simulink model "Model"  (R2023b)
settings: Solver=VariableStepAuto  StartTime=0.0  StopTime=1  RelTol=1e-3
undefined symbols (not defined in the file): D1, Delta
libraries: spsThreePhaseTransformerTwoWindingsLib x4, spsThreePhaseProgrammableVoltageSourceLib x2, spsGroundLib x2, spsDistributedParametersLineLib x2, spsThreePhaseMutualInductanceZ1Z0Lib x2, spsThreePhaseFaultLib x1, spsThreePhaseParallelRLCLoadLib x1, spsThreePhaseVIMeasurementLib x1, sps_lib x1
settings Model: Creator=SJ  LastModifiedBy=SJ

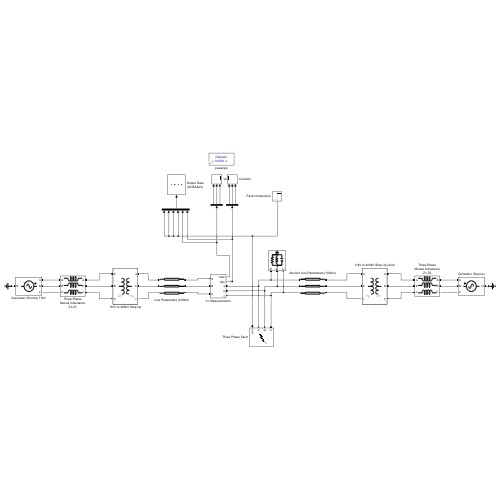
[thumbnail: Simulink's stored preview of the top-level diagram]
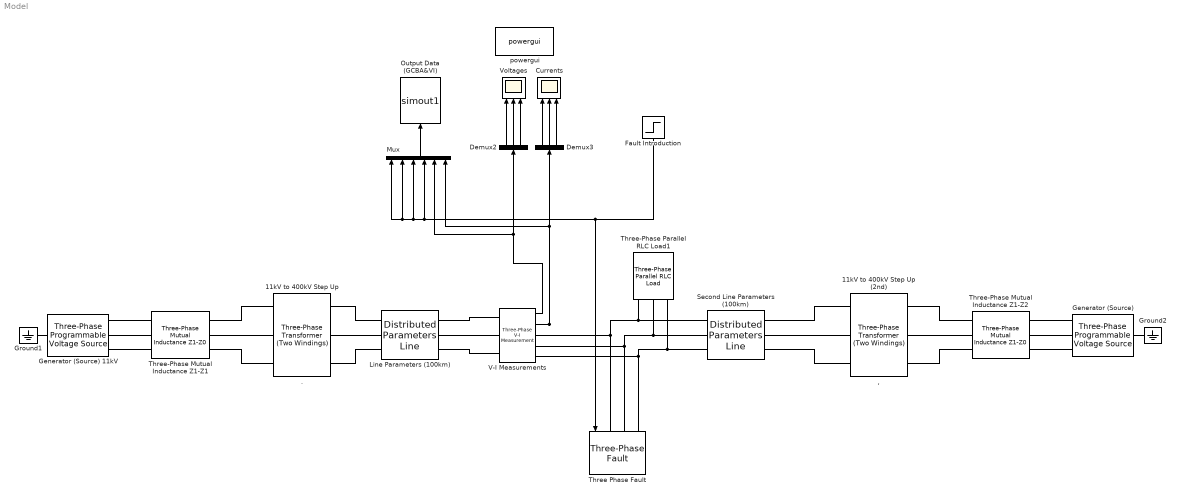
== system Model ==
  , : spsThreePhaseTransformerTwoWindingsLib/Three-Phase Transformer (Two Windings)  Winding1Connection=Delta (D1)  Winding2Connection=Yg  CoreType=Three single-phase transformers  SetSaturation=off  Hysteresis=off  DataFile='hysteresis'  SetInitialFlux=off  Measurements=None  UNITS=pu  NominalPower=[ 2500e3 , 50 ]  Winding1=[ 11e3 , 0.002 , 0.08 ]  Winding2=[ 4e5, 0.002, 0.08 ]  Rm=500  Lm=500  L0=0.5  Saturation=[ 0,0 ; 0.0024,1.2 ; 1.0,1.52 ]  InitialFluxes=[ 0.8 , -0.8 , 0.7 ]  BreakLoop=off  DiscreteSolver=Trapezoidal iterative  DataType=off  TransfoNumber=1
  . : spsThreePhaseTransformerTwoWindingsLib/Three-Phase Transformer (Two Windings)  Winding1Connection=Delta (D1)  Winding2Connection=Yg  CoreType=Three single-phase transformers  SetSaturation=off  Hysteresis=off  DataFile='hysteresis'  SetInitialFlux=off  Measurements=None  UNITS=pu  NominalPower=[ 2500e3 , 50 ]  Winding1=[ 11e3 , 0.002 , 0.08 ]  Winding2=[ 4e5, 0.002, 0.08 ]  Rm=500  Lm=500  L0=0.5  Saturation=[ 0,0 ; 0.0024,1.2 ; 1.0,1.52 ]  InitialFluxes=[ 0.8 , -0.8 , 0.7 ]  BreakLoop=off  DiscreteSolver=Trapezoidal iterative  DataType=off  TransfoNumber=1
  11kV to 400kV Step Up : spsThreePhaseTransformerTwoWindingsLib/Three-Phase Transformer (Two Windings)  Winding1Connection=Delta (D1)  Winding2Connection=Yg  CoreType=Three single-phase transformers  SetSaturation=off  Hysteresis=off  DataFile='hysteresis'  SetInitialFlux=off  Measurements=None  UNITS=pu  NominalPower=[ 2500e3 , 50 ]  Winding1=[ 11e3 , 0.002 , 0.08 ]  Winding2=[ 4e2, 0.002, 0.08 ]  Rm=500  Lm=500  L0=0.5  Saturation=[ 0,0 ; 0.0024,1.2 ; 1.0,1.52 ]  InitialFluxes=[ 0.8 , -0.8 , 0.7 ]  BreakLoop=off  DiscreteSolver=Trapezoidal iterative  DataType=off  TransfoNumber=1
  11kV to 400kV Step Up (2nd) : spsThreePhaseTransformerTwoWindingsLib/Three-Phase Transformer (Two Windings)  Winding1Connection=Delta (D1)  Winding2Connection=Yg  CoreType=Three single-phase transformers  SetSaturation=off  Hysteresis=off  DataFile='hysteresis'  SetInitialFlux=off  Measurements=None  UNITS=pu  NominalPower=[ 2500e3 , 50 ]  Winding1=[ 11e3 , 0.002 , 0.08 ]  Winding2=[ 4e2 , 0.002 , 0.08 ]  Rm=500  Lm=500  L0=0.5  Saturation=[ 0,0 ; 0.0024,1.2 ; 1.0,1.52 ]  InitialFluxes=[ 0.8 , -0.8 , 0.7 ]  BreakLoop=off  DiscreteSolver=Trapezoidal iterative  DataType=off  TransfoNumber=1
  Currents : Scope  NumInputPorts=3
  Demux2 : Demux  Outputs=3
  Demux3 : Demux  Outputs=3
  Fault Introduction : Step  Time=0.1  SampleTime=0
  Generator (Source) : spsThreePhaseProgrammableVoltageSourceLib/Three-Phase Programmable Voltage Source  PositiveSequence="[11e3  0 50]"  VariationEntity=None  VariationType=Table of time-amplitude pairs  VariationTypeAlt=Step  VariationStep=0.5  VariationRate=10  VariationMagnitude=0.3  VariationFrequency=2  VariationTiming=[1 2]  VariationPhaseA=off  Amplitudes=[1 0.8 1.2 1.0]  TimeValues=[0 0.1 0.15 0.2]  HarmonicGeneration=off  HarmonicA=[3 0.2 -25 0]  HarmonicB=[2 0.15 35 2]  Timing="[0.05  3]"  BusType=swing  Pref=0  Qref=0  Qmin=-inf  Qmax=inf
  Generator (Source) 11kV : spsThreePhaseProgrammableVoltageSourceLib/Three-Phase Programmable Voltage Source  PositiveSequence="[11e3  0 50]"  VariationEntity=None  VariationType=Table of time-amplitude pairs  VariationTypeAlt=Step  VariationStep=0.5  VariationRate=10  VariationMagnitude=0.3  VariationFrequency=2  VariationTiming=[1 2]  VariationPhaseA=off  Amplitudes=[1 0.8 1.2 1.0]  TimeValues=[0 0.1 0.15 0.2]  HarmonicGeneration=off  HarmonicA=[3 0.2 -25 0]  HarmonicB=[2 0.15 35 2]  Timing="[0.05  3]"  BusType=swing  Pref=0  Qref=0  Qmin=-inf  Qmax=inf
  Ground1 : spsGroundLib/Ground  LConnTagsString=a
  Ground2 : spsGroundLib/Ground  LConnTagsString=a
  Line Parameters (100km) : spsDistributedParametersLineLib/Distributed Parameters Line  Phases=3  Length=100  Frequency=50  Resistance=[0.01273 0.3864]  Inductance="[0.9337e-3  4.1264e-3]"  Capacitance=[12.74e-9 7.751e-9]  x1=[-0.0006 -4.82329263048478e-14 302.291329147411 -261.391829825195;-0.0005 -4.02670460526195e-14 310.352682416144 -251.767648625029;-0.0004 -3.22614270874366e-14 318.107755056666 -241.895003151946;-0.0003 -2.42239699886876e-14 325.548893748562 -231.78363651509;-0.0002 -1.61626067561552e-14 332.668754986322 -221.443527412571;-0.0001 -8.08529298208965e-15 339.460312326496 -210.884880283698]  x2=[-0.0006 1.07075587974401e-13 258.197390789364 -298.948014119863;-0.0005 1.01302421932401e-13 267.460170011688 -290.690325284424;-0.0004 9.54292826303437e-14 276.458998337068 -282.145760193398;-0.0003 8.94619661476469e-14 285.184995008388 -273.322751300931;-0.0002 8.34063615052364e-14 293.629548520437 -264.230005851586;-0.0001 7.72684448537924e-14 301.784325118421 -254.876497287341]  x3=[-0.0006 3.2797979396176e-15 -0.28191137078804 0.421950096006032;-0.0005 3.29091704997219e-15 -0.295026037352981 0.412886838955771;-0.0004 3.2987884225157e-15 -0.307849548837979 0.403416112443893;-0.0003 3.30340428915374e-15 -0.320369249985401 0.393547262934051;-0.0002 3.30476009458321e-15 -0.332572785361736 0.383290029789229;-0.0001 3.30285450078786e-15 -0.344448111550917 0.372654535660172]  x4=[-0.0006 -3.17636211581e-15 2.23300549703812 -2.5964882734215;-0.0005 -3.15925327302886e-15 2.31346131122797 -2.52506666550988;-0.0004 -3.13902662868852e-15 2.39163401841121 -2.45115312165439;-0.0003 -3.11570214404494e-15 2.46744647156375 -2.37482058559914;-0.0002 -3.08930283754847e-15 2.54082385294727 -2.29614438834146;-0.0001 -3.05985476212738e-15 2.61169374794533 -2.21520217378936]  x5=0.000565541566995743  V1=[2.024e-13 399.6 399.6;314.2 314.2 314.2;-1.932 0.938 -0.6328]  V2=[2.05e-13 395 395;314.2 314.2 314.2;0.8051 0.7925 -0.7783]  I1=[3.039e-15 0.5075 0.5075;314.2 314.2 314.2;-0.08862 -2.472 2.24]  I2=[2.819e-15 3.425 3.425;314.2 314.2 314.2;3.041 0.7904 -0.7804]  nHarmo=1  Measurements=None  Decoupling=off  VsMag0=0  VrMag0=0  VsAngle0=0  VrAngle0=0  IsMag0=0  IrMag0=0  IsAngle0=0  IrAngle0=0
      settings: LibrarySourceBlock=sps_lib/Power Grid Elements/Distributed Parameters Line
  Mux : Mux  Inputs=6
  Output Data (GCBA&VI) : ToWorkspace  VariableName=simout1  SaveFormat=Timeseries  SampleTime=-1
  Second Line Parameters (100km) : spsDistributedParametersLineLib/Distributed Parameters Line  Phases=3  Length=100  Frequency=60  Resistance=[0.01273 0.3864]  Inductance="[0.9337e-3  4.1264e-3]"  Capacitance=[12.74e-9 7.751e-9]  x1=[-0.0006 -1.36928565449085e-13 302.291329147411 -261.391829825195;-0.0005 -1.38135887665828e-13 310.352682416144 -251.767648625028;-0.0004 -1.39206886438792e-13 318.107755056666 -241.895003151946;-0.0003 -1.40140504821492e-13 325.548893748562 -231.78363651509;-0.0002 -1.40935821445302e-13 332.668754986322 -221.443527412571;-0.0001 -1.41592051428733e-13 339.460312326496 -210.884880283698]  x2=[-0.0006 1.07075587974401e-13 258.197390789364 -298.948014119863;-0.0005 1.01302421932401e-13 267.460170011688 -290.690325284424;-0.0004 9.54292826303437e-14 276.458998337068 -282.145760193398;-0.0003 8.94619661476469e-14 285.184995008388 -273.322751300931;-0.0002 8.34063615052364e-14 293.629548520437 -264.230005851586;-0.0001 7.72684448537924e-14 301.784325118421 -254.876497287341]  x3=[-0.0006 1.12667629661657e-15 -0.281911370788044 0.421950096006022;-0.0005 1.11731299989936e-15 -0.295026037352985 0.412886838955761;-0.0004 1.10684705014609e-15 -0.307849548837983 0.403416112443883;-0.0003 1.09528877598558e-15 -0.320369249985405 0.39354726293404;-0.0002 1.082649584039e-15 -0.332572785361739 0.383290029789218;-0.0001 1.06894194766283e-15 -0.34444811155092 0.37265453566016]  x4=[-0.0006 -3.19598852625168e-15 2.23300549703812 -2.59648827342149;-0.0005 -3.24813563146854e-15 2.31346131122797 -2.52506666550987;-0.0004 -3.2970772189693e-15 2.39163401841121 -2.45115312165439;-0.0003 -3.34276498931591e-15 2.46744647156374 -2.37482058559913;-0.0002 -3.38515385419496e-15 2.54082385294727 -2.29614438834145;-0.0001 -3.4242019809145e-15 2.61169374794533 -2.21520217378935]  x5=0.000565541566995742  V1=[3.558e-13 399.6 399.6;314.2 314.2 314.2;-1.251 0.938 -0.6328]  V2=[2.05e-13 395 395;314.2 314.2 314.2;0.8051 0.7925 -0.7783]  I1=[4.38e-15 0.5075 0.5075;314.2 314.2 314.2;0.2418 -2.472 2.24]  I2=[2.604e-15 3.425 3.425;314.2 314.2 314.2;-2.475 0.7904 -0.7804]  nHarmo=1  Measurements=None  Decoupling=off  VsMag0=0  VrMag0=0  VsAngle0=0  VrAngle0=0  IsMag0=0  IrMag0=0  IsAngle0=0  IrAngle0=0
      settings: LibrarySourceBlock=sps_lib/Power Grid Elements/Distributed Parameters Line
  Three Phase Fault : spsThreePhaseFaultLib/Three-Phase Fault  InitialStates=0  FaultA=on  FaultB=on  FaultC=on  GroundFault=off  SwitchTimes=[0.25]  External=on  SwitchStatus=NaN  FaultResistance=0.001  GroundResistance=0.01  SnubberResistance=1e6  SnubberCapacitance=inf  Measurements=None
  Three-Phase Mutual Inductance Z1-Z1 : spsThreePhaseMutualInductanceZ1Z0Lib/Three-Phase Mutual Inductance Z1-Z0  LConnTagsString=a|b|c  RConnTagsString=A|B|C  PositiveSequence="[ 2  50e-3]"  ZeroSequence="[4  100e-3]"
      settings: AttributesFormatString=\n
      settings: LibrarySourceBlock=|
      | sps_lib/Power Grid Elements/Three-Phase
      | Mutual Inductance
      | Z1-Z0
  Three-Phase Mutual Inductance Z1-Z2 : spsThreePhaseMutualInductanceZ1Z0Lib/Three-Phase Mutual Inductance Z1-Z0  LConnTagsString=a|b|c  RConnTagsString=A|B|C  PositiveSequence="[ 2  50e-3]"  ZeroSequence="[4  100e-3]"
      settings: AttributesFormatString=\n
      settings: LibrarySourceBlock=|
      | sps_lib/Power Grid Elements/Three-Phase
      | Mutual Inductance
      | Z1-Z0
  Three-Phase Parallel RLC Load1 : spsThreePhaseParallelRLCLoadLib/Three-Phase Parallel RLC Load  LConnTagsString=A|B|C  Configuration=Y (grounded)  NominalVoltage=1000  Vabc=[1e3 1e3 1e3]  Vabcp=[1e3 1e3 1e3]  NominalFrequency=60  UnbalancedPower=off  ActivePower=10e3  InductivePower=100  CapacitivePower=100  Pabc=[10e3 9e3 11e3]  QLabc=[100 90 110]  QCabc=[100 90 110]  Pabcp=[10e3 9e3 11e3]  QLabcp=[100 90 110]  QCabcp=[100 90 110]  Measurements=None  LoadType=constant Z
  V-I Measurements : spsThreePhaseVIMeasurementLib/Three-Phase V-I Measurement  VoltageMeasurement=phase-to-phase  SetLabelV=off  LabelV=Vabc  Vpu=off  VpuLL=off  CurrentMeasurement=yes  SetLabelI=off  LabelI=Iabc  Ipu=off  Pbase=2500e6  Vbase=400  OutputType=Complex  PhasorSimulation=off  PSBequivalent=0
  Voltages : Scope  NumInputPorts=3
  powergui : sps_lib/powergui  Priority=1  SimulationMode=Discrete  SampleTime=1e-4  frequency=60  Iterations=50  frequencyindice=50  Pbase=100e6  ErrMax=1e-4  UnitsV=kV  UnitsW=MW  buscounter=0  FunctionMessages=off  echomessages=off  EnableUseOfTLC=off  CurrentSourceSwitches=off  DisableSnubberDevices=off  DisableRonSwitches=off  DisableVfSwitches=off  DisplayEquations=off  AutomaticDiscreteSolvers=off  SolverType=Tustin/Backward Euler (TBE)  Interpol=off  ExternalGateDelay=off  methode=off  Ts=100  x0status=blocks  SPID=on  SwTol=0  HookPort=off  NonlinearTolerance=1e-4  nMaxIteration=100  ContinueOnMaxIteration=off  RestoreLinks=warning  ResistiveCurrentMeasurement=off  Frange=[0:2:500]  Ylog=off  Xlog=on  ShowGrid=off  save=off  variable=ZData  structure=0  ZoomFFT=off  StartTime=0.0  cycles=1  DisplayStyle=1  fundamental=60  FreqAxis=off  MaxFrequency=1000  frequencyindicesteady=1  RmsSteady=1  display=off
  wires:
  Demux3/2 -> Currents/2
  Demux3/1 -> Currents/1
  Demux2/1 -> Voltages/1
  Demux3/3 -> Currents/3
  Demux2/2 -> Voltages/2
  Demux2/3 -> Voltages/3
  V-I Measurements/2 -> Mux/6, Demux3/1
  V-I Measurements/1 -> Mux/5, Demux2/1
  Fault Introduction/1 -> Three Phase Fault/1, Mux/4, Mux/3, Mux/1, Mux/2
  Mux/1 -> Output Data (GCBA&VI)/1
  connections:
  V-I Measurements/RConn3 -- Second Line Parameters (100km)/RConn3 -- Three-Phase Parallel RLC Load1/LConn3 -- Three Phase Fault/LConn3
  Second Line Parameters (100km)/RConn2 -- V-I Measurements/RConn2 -- Three Phase Fault/LConn2 -- Three-Phase Parallel RLC Load1/LConn2
  Second Line Parameters (100km)/RConn1 -- V-I Measurements/RConn1 -- Three Phase Fault/LConn1 -- Three-Phase Parallel RLC Load1/LConn1
  Ground1/LConn1 -- Generator (Source) 11kV/LConn1
  Line Parameters (100km)/RConn3 -- V-I Measurements/LConn3
  Line Parameters (100km)/RConn1 -- V-I Measurements/LConn1
  11kV to 400kV Step Up/LConn3 -- Three-Phase Mutual Inductance Z1-Z1/RConn3
  11kV to 400kV Step Up/LConn2 -- Three-Phase Mutual Inductance Z1-Z1/RConn2
  11kV to 400kV Step Up/LConn1 -- Three-Phase Mutual Inductance Z1-Z1/RConn1
  Line Parameters (100km)/RConn2 -- V-I Measurements/LConn2
  Three-Phase Mutual Inductance Z1-Z1/LConn3 -- Generator (Source) 11kV/RConn3
  Generator (Source) 11kV/RConn2 -- Three-Phase Mutual Inductance Z1-Z1/LConn2
  Three-Phase Mutual Inductance Z1-Z1/LConn1 -- Generator (Source) 11kV/RConn1
  Line Parameters (100km)/LConn3 -- 11kV to 400kV Step Up/RConn3
  Line Parameters (100km)/LConn2 -- 11kV to 400kV Step Up/RConn2
  Line Parameters (100km)/LConn1 -- 11kV to 400kV Step Up/RConn1
  Three-Phase Mutual Inductance Z1-Z2/LConn1 -- Generator (Source)/RConn1
  Second Line Parameters (100km)/LConn1 -- 11kV to 400kV Step Up (2nd)/RConn1
  11kV to 400kV Step Up (2nd)/LConn1 -- Three-Phase Mutual Inductance Z1-Z2/RConn1
  Generator (Source)/RConn2 -- Three-Phase Mutual Inductance Z1-Z2/LConn2
  Ground2/LConn1 -- Generator (Source)/LConn1
  Second Line Parameters (100km)/LConn3 -- 11kV to 400kV Step Up (2nd)/RConn3
  11kV to 400kV Step Up (2nd)/LConn2 -- Three-Phase Mutual Inductance Z1-Z2/RConn2
  Second Line Parameters (100km)/LConn2 -- 11kV to 400kV Step Up (2nd)/RConn2
  11kV to 400kV Step Up (2nd)/LConn3 -- Three-Phase Mutual Inductance Z1-Z2/RConn3
  Three-Phase Mutual Inductance Z1-Z2/LConn3 -- Generator (Source)/RConn3
